simulink model "sampleModel1933_4_sub_sub_sub"  (R2023a)
settings: Solver=VariableStepAuto  StartTime=0.0  StopTime=10.0  RelTol=1e-3
libraries: hdlsllib x5, simulink x2
settings Model: Creator=user1  LastModifiedBy=user1
settings OptimizationCC: BlockReduction=off  ConditionallyExecuteInputs=off

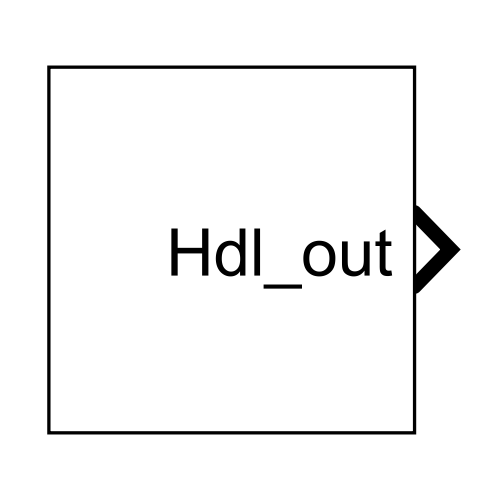
[thumbnail: Simulink's stored preview of the top-level diagram]
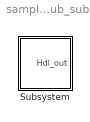
== system sampleModel1933_4_sub_sub_sub ==
  Subsystem : Subsystem

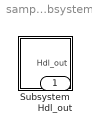
== system sampleModel1933_4_sub_sub_sub/Subsystem ==
  Subsystem : Subsystem
  Hdl_out : Outport  OutDataTypeStr=uint8

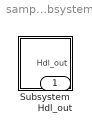
== system sampleModel1933_4_sub_sub_sub/Subsystem/Subsystem ==
  Subsystem : Subsystem
  Hdl_out : Outport  OutDataTypeStr=uint8

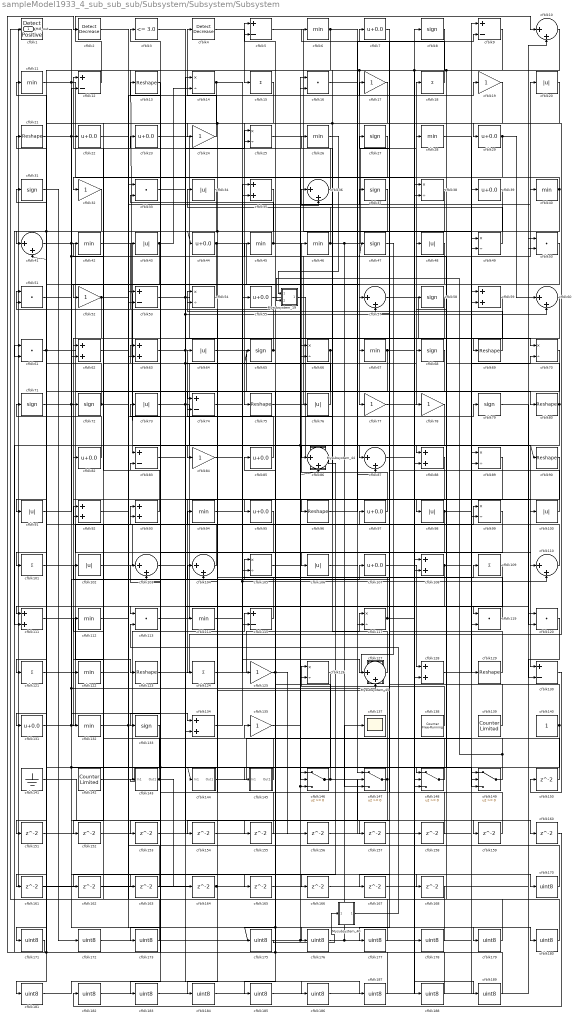
== system sampleModel1933_4_sub_sub_sub/Subsystem/Subsystem/Subsystem ==
  Mysubsystem_19 : Subsystem  TreatAsAtomicUnit=on  RTWFcnName=Mysubsystem_19
      settings: RTWFcnNameOpts=User specified  RTWFileNameOpts=Use function name
  Mysubsystem_40 : Subsystem  TreatAsAtomicUnit=on  RTWFcnName=Mysubsystem_40
      settings: RTWFcnNameOpts=User specified  RTWFileNameOpts=Use function name
  Mysubsystem_44 : Subsystem  TreatAsAtomicUnit=on  RTWFcnName=Mysubsystem_44
      settings: RTWFcnNameOpts=User specified  RTWFileNameOpts=Use function name
  Mysubsystem_45 : Subsystem  TreatAsAtomicUnit=on  RTWFcnName=Mysubsystem_45
      settings: RTWFcnNameOpts=User specified  RTWFileNameOpts=Use function name
  cfblk1 : hdlsllib/Logic and Bit Operations/Detect Rise Positive  vinit=0  OutDataTypeStr=uint8
  cfblk{10,36,41,57,60,86..87,103..104,110,127} (11 alike) : Sum  Inputs=|++  OutDataTypeStr=uint8
  cfblk{20,34,43,48,64,73,76,91,98,100,102,106} (12 alike) : Abs  OutDataTypeStr=uint8  SaturateOnIntegerOverflow=off
  cfblk{15,18,101,109,121,124} (6 alike) : Sum  Inputs=+  OutDataTypeStr=uint8
  cfblk{14,25,38,49,54,66,70,89,99,105,117,126} (12 alike) : Product  Inputs=*/  OutDataTypeStr=uint8  RndMeth=Zero  SaturateOnIntegerOverflow=on
  cfblk{7,22..23,29,39,44,55,82,85,95,97,107,131} (13 alike) : Bias  Bias=0.0  SaturateOnIntegerOverflow=off
  cfblk{35,59,62..63,88,92..93,108,111,128,134} (11 alike) : Sum  OutDataTypeStr=uint8
  cfblk{6,11,26,28,40,42,45..46,67,94,112,114,122,132} (14 alike) : MinMax  OutDataTypeStr=uint8
  cfblk{16,33,50..51,61,113,119..120} (8 alike) : DotProduct  OutDataTypeStr=uint8
  cfblk{5,9,12,53,74,83,115,130} (8 alike) : Sum  Inputs=+-  OutDataTypeStr=uint8
  cfblk{13,21,69,75,80,90,96,123,129} (9 alike) : Reshape
  cfblk{17,19,24,32,52,77..78,84,125,135} (10 alike) : Gain  OutDataTypeStr=uint8
  cfblk{8,27,31,37,47,58,65,68,71..72,79,133} (12 alike) : Signum
  cfblk137 : Scope
  cfblk138 : hdlsllib/Sources/Counter Free-Running  NumBits=16  tsamp=-1
  cfblk139 : hdlsllib/Sources/Counter Limited  uplimit=7  tsamp=-1
  cfblk140 : Constant  OutDataTypeStr=uint8  SampleTime=-1
  cfblk141 : Ground
  cfblk142 : hdlsllib/Sources/Counter Limited  uplimit=7  tsamp=-1
  cfblk143 : Subsystem
      settings: LibrarySourceBlock=|
      | hdlsllib/Ports &
      | Subsystems/Subsystem
  cfblk144 : Subsystem
      settings: LibrarySourceBlock=|
      | hdlsllib/Ports &
      | Subsystems/Subsystem
  cfblk145 : Subsystem
      settings: LibrarySourceBlock=|
      | hdlsllib/Ports &
      | Subsystems/Subsystem
  cfblk{146..149} (4 alike) : Switch  OutDataTypeStr=uint8  SaturateOnIntegerOverflow=off  InputSameDT=off
  cfblk{150..168} (19 alike) : Delay  SampleTime=1
  cfblk{170..173,175..189} (19 alike) : DataTypeConversion  OutDataTypeStr=uint8  SaturateOnIntegerOverflow=off  RndMeth=Floor
  cfblk2 : simulink/Logic and Bit Operations/Detect Decrease  vinit=0.0  OutDataTypeStr=uint8
      settings: LibrarySourceBlock=|
      | hdlsllib/Logic and Bit
      | Operations/Detect
      | Decrease
  cfblk3 : hdlsllib/Logic and Bit Operations/Compare To Constant  relop=<=  const=3.0  OutDataTypeStr=uint8
  cfblk4 : simulink/Logic and Bit Operations/Detect Decrease  vinit=0.0  OutDataTypeStr=uint8
      settings: LibrarySourceBlock=|
      | hdlsllib/Logic and Bit
      | Operations/Detect
      | Decrease
  Hdl_out : Outport  OutDataTypeStr=uint8
  wires:
  cfblk142/1 -> cfblk115/1
  cfblk41/1 -> cfblk148/3, cfblk106/1
  cfblk71/1 -> cfblk134/1, cfblk107/1
  cfblk123/1 -> cfblk29/1
  cfblk32/1 -> cfblk61/2, cfblk111/1
  cfblk40/1 -> cfblk53/2, cfblk32/1
  cfblk104/1 -> cfblk11/1
  cfblk89/1 -> cfblk124/1
  cfblk8/1 -> cfblk134/2, cfblk77/1
  cfblk77/1 -> cfblk18/1
  cfblk146/1 -> cfblk160/1, cfblk25/2
  cfblk97/1 -> cfblk46/1
  cfblk107/1 -> cfblk128/1
  cfblk115/1 -> cfblk51/1
  cfblk11/1 -> cfblk128/2, cfblk159/1, cfblk127/2
  cfblk43/1 -> cfblk14/2, cfblk101/1
  cfblk113/1 -> cfblk68/1
  cfblk75/1 -> cfblk20/1
  cfblk131/1 -> cfblk149/3, cfblk104/1, cfblk105/1
  cfblk33/1 -> cfblk176/1
  cfblk36/1 -> cfblk12/1
  cfblk19/1 -> cfblk75/1
  cfblk5/1 -> cfblk147/1
  cfblk9/1 -> cfblk98/1, cfblk148/2, cfblk83/1
  cfblk111/1 -> cfblk123/1
  cfblk34/1 -> cfblk131/1
  cfblk54/1 -> cfblk52/1
  cfblk46/1 -> cfblk5/2, cfblk147/3, cfblk28/1
  cfblk52/1 -> cfblk149/2, cfblk82/1
  cfblk57/1 -> cfblk69/1
  cfblk4/1 -> cfblk15/1
  cfblk138/1 -> cfblk126/1
  cfblk110/1 -> cfblk23/1
  cfblk25/1 -> cfblk59/1
  cfblk58/1 -> cfblk72/1
  cfblk121/1 -> cfblk97/1
  cfblk85/1 -> cfblk64/1
  cfblk21/1 -> cfblk180/1, cfblk66/1
  cfblk127/1 -> cfblk76/1
  cfblk68/1 -> cfblk185/1, cfblk175/1
  cfblk95/1 -> cfblk133/1
  cfblk122/1 -> cfblk99/1
  cfblk28/1 -> cfblk80/1
  cfblk148/1 -> cfblk94/1
  cfblk101/1 -> cfblk93/1
  cfblk53/1 -> cfblk45/1, cfblk146/1
  cfblk90/1 -> cfblk95/1
  cfblk80/1 -> cfblk48/1, cfblk111/2
  cfblk42/1 -> cfblk130/1
  cfblk15/1 -> cfblk62/2, cfblk44/1, cfblk84/1
  cfblk27/1 -> cfblk62/1
  cfblk23/1 -> cfblk78/1
  cfblk88/1 -> cfblk132/1
  cfblk119/1 -> cfblk93/2
  cfblk94/1 -> cfblk119/1
  cfblk91/1 -> cfblk47/1, cfblk12/2
  cfblk24/1 -> cfblk4/1
  cfblk98/1 -> cfblk104/2, cfblk39/1
  cfblk139/1 -> cfblk102/1
  cfblk60/1 -> cfblk148/1
  cfblk20/1 -> cfblk24/1
  cfblk103/1 -> cfblk187/1
  cfblk128/1 -> cfblk59/2
  cfblk114/1 -> cfblk40/1
  cfblk12/1 -> cfblk10/1
  cfblk102/1 -> cfblk35/1
  cfblk69/1 -> cfblk54/1
  cfblk124/1 -> cfblk117/1
  cfblk61/1 -> cfblk41/2, cfblk126/2
  cfblk14/1 -> cfblk122/1, cfblk110/2, cfblk127/1
  cfblk76/1 -> cfblk22/1
  cfblk70/1 -> cfblk121/1
  cfblk133/1 -> cfblk143/1(In1)
  cfblk145/1(Out1) -> cfblk135/1
  cfblk63/1 -> cfblk70/1, cfblk100/1
  cfblk29/1 -> cfblk60/1, cfblk35/2
  cfblk84/1 -> cfblk55/1
  cfblk66/1 -> cfblk146/2, cfblk36/1
  cfblk135/1 -> cfblk17/1
  cfblk134/1 -> cfblk109/1
  cfblk67/1 -> cfblk105/2, cfblk8/1
  cfblk140/1 -> cfblk145/1(In1), cfblk92/1
  cfblk10/1 -> cfblk96/1
  cfblk120/1 -> cfblk130/2
  cfblk147/1 -> cfblk154/1, cfblk74/2
  cfblk6/1 -> cfblk171/1, cfblk88/1
  cfblk125/1 -> cfblk156/1, cfblk155/1
  cfblk143/1(Out1) -> cfblk164/1, cfblk92/2
  cfblk7/1 -> cfblk87/1
  cfblk105/1 -> cfblk16/1
  cfblk96/1 -> cfblk9/2
  cfblk132/1 -> cfblk165/1, cfblk37/1
  cfblk117/1 -> cfblk189/1, cfblk63/1
  cfblk16/1 -> cfblk108/2
  cfblk86/1 -> cfblk26/1
  cfblk65/1 -> cfblk5/1, cfblk43/1
  cfblk93/1 -> cfblk42/1
  cfblk144/1(Out1) -> cfblk89/2
  cfblk18/1 -> cfblk7/1
  cfblk74/1 -> cfblk125/1
  cfblk126/1 -> cfblk173/1, cfblk161/1
  cfblk73/1 -> cfblk87/2, cfblk114/1
  cfblk92/1 -> cfblk79/1
  cfblk39/1 -> cfblk41/1
  cfblk129/1 -> cfblk27/1
  cfblk17/1 -> cfblk91/1, cfblk86/1
  cfblk72/1 -> cfblk19/1, cfblk51/2
  cfblk79/1 -> cfblk120/1
  cfblk49/1 -> cfblk34/1
  cfblk82/1 -> cfblk21/1
  cfblk31/1 -> cfblk172/1
  cfblk45/1 -> cfblk13/1, cfblk90/1, cfblk86/2
  cfblk64/1 -> cfblk129/1
  cfblk106/1 -> cfblk120/2
  cfblk3/1 -> cfblk115/2
  cfblk1/1 -> cfblk57/1
  cfblk83/1 -> cfblk65/1, cfblk60/2, cfblk25/1
  cfblk149/1 -> cfblk3/1, Mysubsystem_19/2(In2)
  cfblk44/1 -> cfblk113/1, cfblk117/2
  cfblk55/1 -> cfblk67/1
  cfblk22/1 -> cfblk110/1
  cfblk37/1 -> cfblk74/1
  cfblk100/1 -> cfblk6/1
  cfblk51/1 -> cfblk168/1, cfblk144/1(In1)
  cfblk108/1 -> cfblk151/1, cfblk70/2
  cfblk130/1 -> cfblk150/1
  cfblk150/1 -> cfblk9/1
  cfblk151/1 -> cfblk14/1
  cfblk35/1 -> cfblk152/1
  cfblk152/1 -> cfblk108/1
  cfblk48/1 -> cfblk153/1
  cfblk153/1 -> cfblk36/2
  cfblk154/1 -> cfblk99/2
  cfblk155/1 -> cfblk54/2
  cfblk156/1 -> cfblk147/2
  cfblk59/1 -> cfblk157/1
  cfblk157/1 -> cfblk49/1
  cfblk158/1 -> cfblk83/2
  cfblk159/1 -> cfblk57/2
  cfblk161/1 -> cfblk66/2
  cfblk162/1 -> cfblk63/2
  cfblk13/1 -> cfblk163/1
  cfblk163/1 -> cfblk53/1
  cfblk164/1 -> Hdl_out/1, cfblk149/1
  cfblk165/1 -> cfblk88/2
  cfblk62/1 -> cfblk166/1
  cfblk166/1 -> cfblk10/2
  cfblk109/1 -> cfblk167/1
  cfblk167/1 -> cfblk89/1
  cfblk168/1 -> cfblk1/1
  cfblk2/1 -> cfblk170/1
  cfblk170/1 -> cfblk73/1
  cfblk171/1 -> cfblk2/1
  cfblk172/1 -> cfblk119/2, cfblk16/2, cfblk146/3
  cfblk173/1 -> cfblk31/1
  cfblk176/1 -> cfblk137/1, cfblk158/1
  cfblk78/1 -> cfblk177/1
  cfblk177/1 -> cfblk33/1
  cfblk87/1 -> cfblk178/1
  cfblk178/1 -> cfblk33/2
  cfblk112/1 -> cfblk179/1
  cfblk179/1 -> cfblk58/1
  cfblk180/1 -> cfblk112/1
  cfblk38/1 -> cfblk181/1
  cfblk160/1 -> cfblk182/1
  cfblk182/1 -> cfblk38/1
  cfblk99/1 -> cfblk183/1
  cfblk183/1 -> cfblk38/2
  cfblk50/1 -> cfblk184/1
  cfblk184/1 -> cfblk49/2
  cfblk185/1 -> cfblk50/1
  cfblk181/1 -> cfblk186/1
  cfblk186/1 -> cfblk50/2
  cfblk187/1 -> cfblk85/1, cfblk61/1, cfblk71/1
  cfblk141/1 -> cfblk188/1
  cfblk188/1 -> cfblk103/1
  cfblk189/1 -> cfblk103/2
  cfblk26/1 -> Mysubsystem_19/1(In1)
  cfblk175/1 -> Mysubsystem_40/1(In1)
  Mysubsystem_40/1(Out1) -> cfblk113/2
  Mysubsystem_19/1(Out1) -> Mysubsystem_44/1(In1)
  Mysubsystem_44/1(Out1) -> cfblk162/1
  cfblk47/1 -> Mysubsystem_45/1(In1)

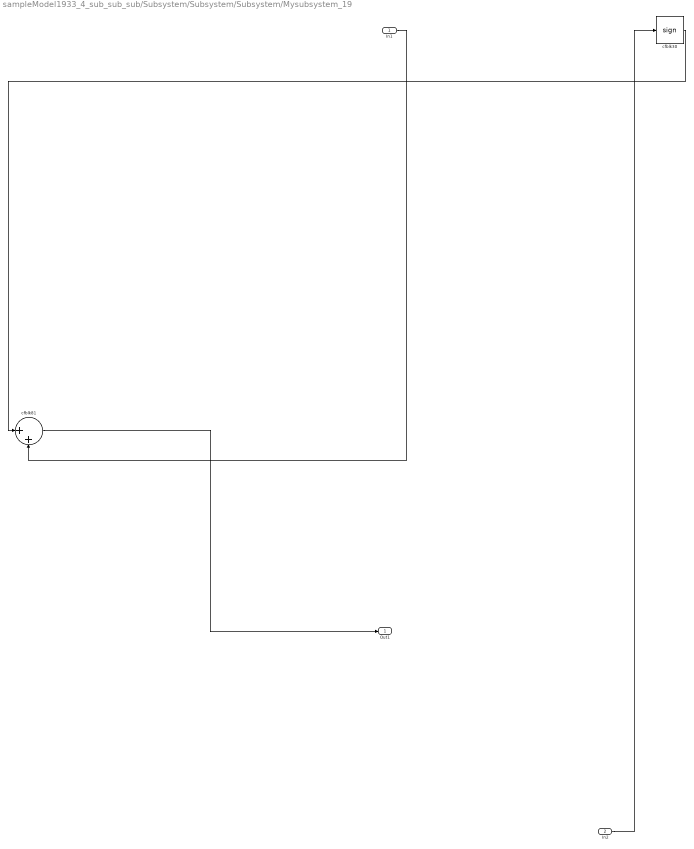
== system sampleModel1933_4_sub_sub_sub/Subsystem/Subsystem/Subsystem/Mysubsystem_19 ==
  In1 : Inport
  In2 : Inport  Port=2
  cfblk30 : Signum
  cfblk81 : Sum  Inputs=|++
  Out1 : Outport
  wires:
  In1/1 -> cfblk81/2
  cfblk81/1 -> Out1/1
  In2/1 -> cfblk30/1
  cfblk30/1 -> cfblk81/1

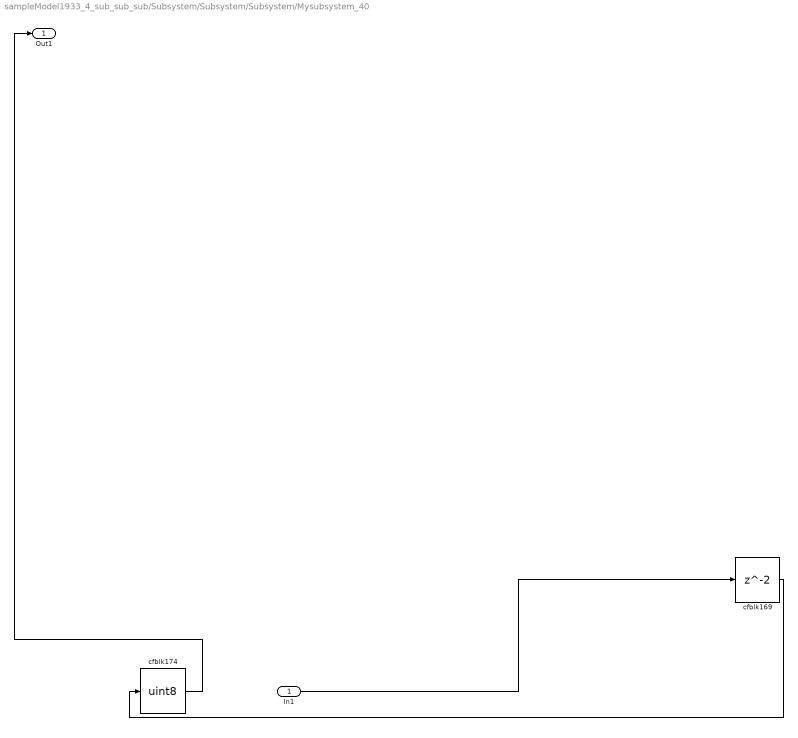
== system sampleModel1933_4_sub_sub_sub/Subsystem/Subsystem/Subsystem/Mysubsystem_40 ==
  In1 : Inport
  cfblk169 : Delay  SampleTime=1
  cfblk174 : DataTypeConversion  OutDataTypeStr=uint8  SaturateOnIntegerOverflow=off  RndMeth=Floor
  Out1 : Outport
  wires:
  cfblk174/1 -> Out1/1
  In1/1 -> cfblk169/1
  cfblk169/1 -> cfblk174/1

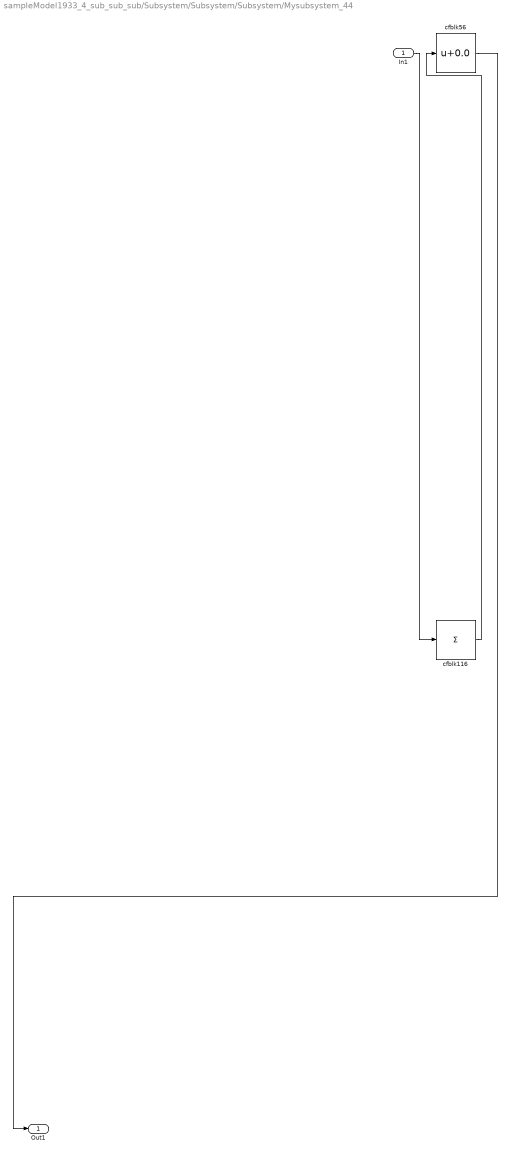
== system sampleModel1933_4_sub_sub_sub/Subsystem/Subsystem/Subsystem/Mysubsystem_44 ==
  In1 : Inport
  cfblk116 : Sum  Inputs=+
  cfblk56 : Bias  Bias=0.0  SaturateOnIntegerOverflow=off
  Out1 : Outport
  wires:
  cfblk56/1 -> Out1/1
  In1/1 -> cfblk116/1
  cfblk116/1 -> cfblk56/1

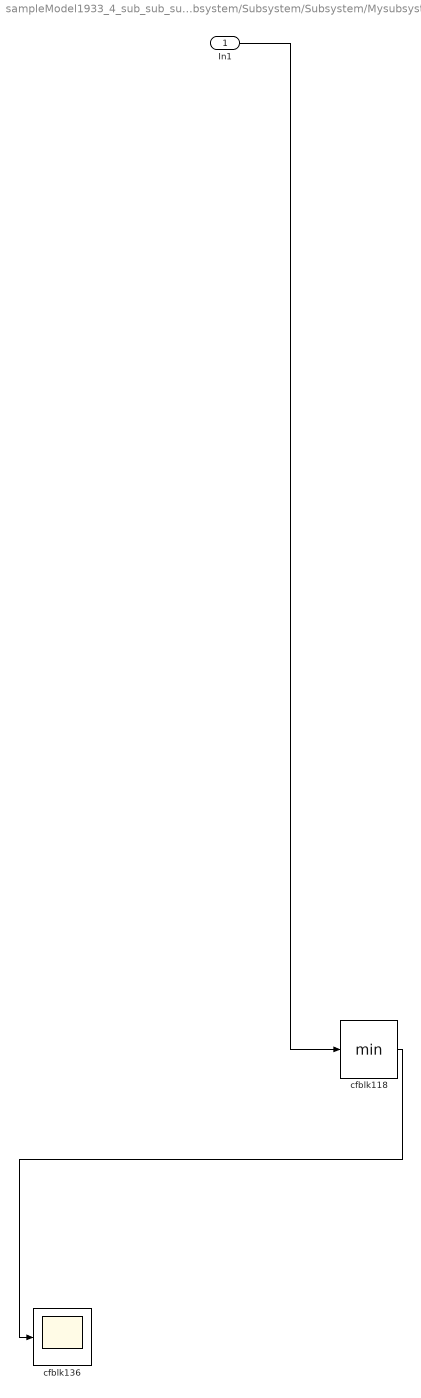
== system sampleModel1933_4_sub_sub_sub/Subsystem/Subsystem/Subsystem/Mysubsystem_45 ==
  In1 : Inport
  cfblk118 : MinMax
  cfblk136 : Scope
  wires:
  In1/1 -> cfblk118/1
  cfblk118/1 -> cfblk136/1

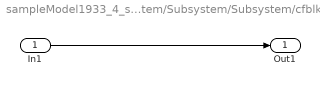
== system sampleModel1933_4_sub_sub_sub/Subsystem/Subsystem/Subsystem/cfblk143 ==
  In1 : Inport
  Out1 : Outport
  wires:
  In1/1 -> Out1/1

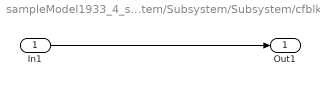
== system sampleModel1933_4_sub_sub_sub/Subsystem/Subsystem/Subsystem/cfblk144 ==
  In1 : Inport
  Out1 : Outport
  wires:
  In1/1 -> Out1/1

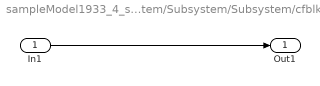
== system sampleModel1933_4_sub_sub_sub/Subsystem/Subsystem/Subsystem/cfblk145 ==
  In1 : Inport
  Out1 : Outport
  wires:
  In1/1 -> Out1/1
